simulink model "TASK3_LAB"  (R2024b)
settings: Solver=ode4  StartTime=0.0  StopTime=T_SIM  FixedStep=T_s  RelTol=1e-3
values from neighbouring files (symbols this model uses):
  control_par = control_par1    [TASK1_LAB_Script.m]    (also in TASK2_LAB_SCRIPT.m = control_par4; TASK2_Scirpt.m = update_control_par(controller_index))
  controller_index = 2    [TASK2_LAB_SCRIPT.m]    (also in TASK2_Scirpt.m = 3)
  d = d_actual    (= 0.1604)    [TASK1_LAB_Script.m]    (also in TASK2_LAB_SCRIPT.m; TASK2_Scirpt.m)
  D = diag([0.8e-3, 0.8e-3, 5e-3, 0.0175/6, 0.0175/6, 0.0175/6*T_s, 0.0175/6*T_s].^2)    [TASK1_LAB_Script.m]    (also in TASK2_LAB_SCRIPT.m; TASK2_Scirpt.m)
  d_actual = 0.16040    (= 0.1604)    [TASK1_LAB_Script.m]    (also in TASK2_LAB_SCRIPT.m; TASK2_Scirpt.m)
  H_enc = [0, 0, 0, 1, 0, 0, 0 ... (first row only)    [TASK1_LAB_Script.m]    (also in TASK2_LAB_SCRIPT.m; TASK2_Scirpt.m)
  H_gyro = [0, 0, 0, 0, 0, -r_actual/d_actual, r_actual/d_actual]    [TASK1_LAB_Script.m]    (also in TASK2_LAB_SCRIPT.m; TASK2_Scirpt.m)
  H_motion_cap = [1, 0, 0, 0, 0, 0, 0 ... (first row only)    [TASK1_LAB_Script.m]    (also in TASK2_LAB_SCRIPT.m; TASK2_Scirpt.m)
  omega_M = 8    [TASK1_LAB_Script.m]    (also in TASK2_LAB_SCRIPT.m = 10; TASK2_Scirpt.m = 10)
  P_INIT_EKF = diag([0.1, 0.1, 0.2, 0.0175/6, 0.0175/6, 0.0175/6*T_s, 0.0175/6*T_s].^2)    [TASK1_LAB_Script.m]    (also in TASK2_LAB_SCRIPT.m; TASK2_Scirpt.m)
  PHI_INIT = [0;0]    [TASK1_LAB_Script.m]    (also in TASK2_LAB_SCRIPT.m; TASK2_Scirpt.m)
  Q_INIT = [-2.2; 0.7; -pi/2]    [TASK1_LAB_Script.m]    (also in TASK2_LAB_SCRIPT.m = [-1.6;-1.1;0]; TASK2_Scirpt.m = [-1.62033177494552;-1.09995932026211;-0.0877488080877385])
  r = r_actual    (= 0.03293)    [TASK1_LAB_Script.m]    (also in TASK2_LAB_SCRIPT.m; TASK2_Scirpt.m)
  R_3 = diag(([sigma_motion_capture, sigma_motion_capture, sigma_motion_capture,               sigma_enc, sigma_enc, sigma_imu]).^2)    [TASK1_LAB_Script.m]    (also in TASK2_LAB_SCRIPT.m; TASK2_Scirpt.m)
  r_actual = 0.03293    [TASK1_LAB_Script.m]    (also in TASK2_LAB_SCRIPT.m; TASK2_Scirpt.m)
  T_s = 0.04    [TASK1_LAB_Script.m]    (also in TASK2_LAB_SCRIPT.m; TASK2_Scirpt.m)
  Z_INIT_EKF = [Q_INIT; 0; 0; 0; 0]    [TASK1_LAB_Script.m]    (also in TASK2_LAB_SCRIPT.m; TASK2_Scirpt.m)
undefined symbols (not defined in the file or in its folder): p_loss, X, Y
libraries: robotlib x6, sharedtransform x2
(part 2 of 2)

== matlab function TASK3_LAB/Actual System/ros/Subsystem/  ==
  data: y output; pos input; condition output
function [y, condition] = check(pos)

x1 = -2.9; y1 = -1.5;
x2 = -1.6; y2 = -1.1;
x3 = -1.5; y3 = -0.7;
x4 = -1.4; y4 = -0.3;
x5 = -0.6; y5 =  0.1;
x6 =  0.2; y6 =  1.5;
x7 =  1.0;
x8 =  1.1;
x9 =  2.9;

P_loss = 0.9;


if ((pos(1) >= x5) && (pos(1) <= x6)) && ((pos(2) >= y1) && (pos(2) <= y5))
    % add noise
    y = pos + 0.02*randn(3,1);
    condition = 1;
elseif ((pos(1) >= x7) && (pos(1) <= x9)) && ((pos(2) >= y1) && (pos(2) <= y6))
    % measurement loss
    if rand > P_loss
        y = pos;
    else
        y = 0*pos;
    end
    condition = 2;
else
    y = pos;
    condition = 0;
end

== matlab function TASK3_LAB/Localizzazione EKF/MATLAB Function ==
  data: P_filt input; P_new output; z_filt input; z_new output; u input; y_new input; D parameter; T_s parameter; r_actual parameter; d_actual parameter; H_enc parameter; H_gyro parameter; H_motion_cap parameter; R_3 parameter; q_EKF output; outlier_flags output
function [P_new, z_new, q_EKF, outlier_flags] = EKF_filtering(P_filt, z_filt, u, y_new, D, T_s, r_actual, d_actual, H_enc, H_gyro, H_motion_cap, R_3)

    % Def state z_filt: [xk , yk , thetak , delta_phi_L_km1 , delta_phi_R_km1 , wLk , wRk ]

    r = r_actual;
    d = d_actual;
    outlier_flags = [0; 0; 0];
        
    % Extraction variables
    x_k = z_filt(1);
    y_k = z_filt(2);
    theta_k = z_filt(3);
    delta_phi_L_km1 = z_filt(4);
    delta_phi_R_km1 = z_filt(5); 
    wL_k = z_filt(6);               % estimate wheels velocities
    wR_k = z_filt(7);
    
    uL_k = u(1);                    % actual wheels velocities (from command input v,w)
    uR_k = u(2);

    % ----------------------

    % PREDICT STEP
    v_k = (r/2) * (wL_k + wR_k);
    omega_k = (r/d) * (wR_k - wL_k);
    theta_mean = theta_k + (omega_k * T_s) / 2;
        
    % State Prediction (approximation with RK2)
    x_kp1 = x_k + v_k * T_s * cos(theta_mean);
    y_kp1 = y_k + v_k * T_s * sin(theta_mean);
    theta_kp1 = theta_k + omega_k * T_s;

    theta_kp1 = atan2(sin(theta_kp1), cos(theta_kp1));
    
    delta_phi_L_k = wL_k * T_s;
    delta_phi_R_k = wR_k * T_s;
    
    wL_kp1 = uL_k; 
    wR_kp1 = uR_k;
    
    z_hat = [x_kp1; y_kp1; theta_kp1; delta_phi_L_k; delta_phi_R_k; wL_kp1; wR_kp1];
    
    % F derivation
    F = zeros(7,7);
    
    F(1,1) = 1;
    F(1, 3) = -T_s * v_k * sin(theta_mean);
    F(1, 6) = (T_s * r / 2) * cos(theta_mean) - v_k * T_s * sin(theta_mean) * (-T_s * r / (2 * d));
    F(1, 7) = (T_s * r / 2) * cos(theta_mean) - v_k * T_s * sin(theta_mean) * (T_s * r / (2 * d));
    
    F(2,2) = 1;
    F(2, 3) = v_k * T_s * cos(theta_mean);
    F(2, 6) = (T_s * r / 2) * sin(theta_mean) + v_k * T_s * cos(theta_mean) * (-T_s * r / (2 * d));
    F(2, 7) = (T_s * r / 2) * sin(theta_mean) + v_k * T_s * cos(theta_mean) * (T_s * r / (2 * d));

    F(3,3) = 1;
    F(3, 6) = -T_s * r / d;
    F(3, 7) = T_s * r / d;

    F(4, 6) = T_s;
    F(5, 7) = T_s;
    
    % Covariance Prediction
    P_hat = F * P_filt * F' + D;
    
    % ----------------------

    % UPDATE STEP
    % H and R will depend on the measurement data y_new and Test_case

    % enc_values (delta_phi)
    % IMU_values (w_gyro)
    % Motion_capture (state q)

    % y_new = [x; y; theta; delta_phi_L; delta_phi_R; omega_gyro]

    %% OBSERVATION MATRIX H ALWAYS FULL (6X7) AND ALSO Y_NEW (6X1) 
    H_full = [H_motion_cap; H_enc; H_gyro];
    y_meas = y_new; 
    
    % Start with full matrix R_3 
    R_current = R_3;
    INFINITY_VAR = 1e9; % Infinite var to put down the Kalman gain

    % IMU not available
    R_current(6,6) = INFINITY_VAR;
    
    % % TEST 3: all active, possibile data loss
    % if norm(y_new(1:3)) < 0.05  
    %     R_current(1,1) = INFINITY_VAR; 
    %     R_current(2,2) = INFINITY_VAR; 
    %     R_current(3,3) = INFINITY_VAR;
    % end
    % 
    % Innovation e_pred
    y_hat = H_full * z_hat;
    e_kp1 = y_meas - y_hat;

    e_kp1(3) = atan2(sin(e_kp1(3)), cos(e_kp1(3)));

    % --- REIEZIONE OUTLIER (INNOVATION GATING) ---

    if norm(y_new(1:3)) < 0.05  
        R_current(1,1) = INFINITY_VAR; 
        R_current(2,2) = INFINITY_VAR; 
        R_current(3,3) = INFINITY_VAR;
    end

    % if isnan(e_kp1(1)) || abs(e_kp1(1)) > 0.08
    %     R_current(1,1) = INFINITY_VAR;
    %     outlier_flags(1) = 1; % Segnala anomalia su X
    % end
    % if isnan(e_kp1(2)) || abs(e_kp1(2)) > 0.08
    %     R_current(2,2) = INFINITY_VAR;
    %     outlier_flags(2) = 1; % Segnala anomalia su Y
    % end
    % 
    % % Threshold Theta (0.15 rad)
    % if isnan(e_kp1(3)) || abs(e_kp1(3)) > 0.15
    %     R_current(3,3) = INFINITY_VAR;
    %     outlier_flags(3) = 1; % Segnala anomalia su Theta
    % end



    
    % Kalman Gain K_pred
    K = P_hat * H_full' / (H_full * P_hat * H_full' + R_current);   
    
    % State and Covariance Update
    z_new = z_hat + K * e_kp1;

    z_new(3) = atan2(sin(z_new(3)), cos(z_new(3)));
    
    P_new = P_hat - K * H_full * P_hat;


    q_EKF = z_new(1:3);

end

== matlab function TASK3_LAB/Planning/Trajectory Planning ==
  data: t input; q_d output; dq_d output; u_DF output; T_circ parameter
function [q_d, dq_d, u_DF] = get_circualt_traj_TASK3(t, T_circ)
   
    % center
    x_c = 2.0;     % x10-x9 /2
    y_c = 0.0;

    x7 = 1.00;
    x8 = 1.45;
    y4 = -0.30;

    
    % Raggio e angolo iniziale (calcolati dal punto di partenza)
    r = sqrt((x8 - x_c)^2 + (y4 - y_c)^2);
    phi0 = atan2(y4 - y_c, x8 - x_c);

    % theta_start = phi0 + pi/2;   % orientation tangent to the circle in (x8,y4)


    % LINE TRAJ
    if t < T_line
    d  = x8 - x7;           % distanza = 0.45 m
    vd = d / T_line;         % velocità costante

    x_d = x7 + vd * t;
    % theta_d = 0 (punta a destra, uguale a theta_robot iniziale → errore zero!)

    q_d  = [x_d; y4; 0];
    dq_d = [vd; 0; 0];
    u_DF = [vd; 0];
   
        
    else 
       
        % 1.5 giri = 3*pi rad in T_trj secondi
        omega = 3 * pi / T_circ;   % constant ang vel

        t_c         = min(t - T_line, T_circ);
        theta_prime = omega * t_c;
        phi         = phi0 + theta_prime;

        q_d  = [x_c + r*cos(phi);
                y_c + r*sin(phi);
                phi + pi/2];

        dq_d = [-omega*r*sin(phi);
                 omega*r*cos(phi);
                 omega];

        u_DF = [omega*r; omega];
    end
end
